simulink library "Addition_library"  (R2022b)
settings: Solver=VariableStepAuto  StartTime=0.0  StopTime=10.0  RelTol=1e-3
settings Model: Creator=Dell  LastModifiedBy=Dell

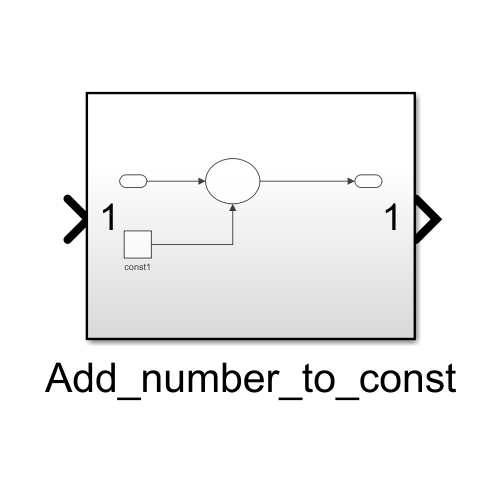
[thumbnail: Simulink's stored preview of the top-level diagram]
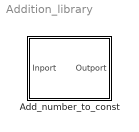
== system Addition_library ==
  Add_number_to_const : Subsystem

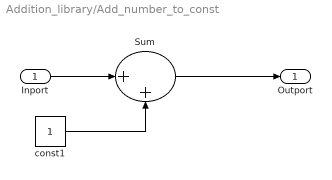
== system Addition_library/Add_number_to_const ==
  Inport : Inport
  Sum : Sum  Inputs=|++
  const1 : Constant
  Outport : Outport
  wires:
  const1/1 -> Sum/2
  Sum/1 -> Outport/1
  Inport/1 -> Sum/1
